simulink model "Auto_pilot"  (R2022a)
settings: Solver=VariableStepAuto  StartTime=0.0  StopTime=10  MaxStep=0.001  RelTol=1e-3
values from neighbouring files (symbols this model uses):
  a_phi1 = -1 * 0.5 * rho * Va^2 * S * b * C_pp * b / (2 * Va)    [Lateral_Autopilot.m]
  a_phi2 = 1 * 0.5 * rho * Va^2 * S * b * C_pa    [Lateral_Autopilot.m]
  k_d_phi = (2 * zeta_phi * w_n_phi - a_phi1) / a_phi2    [Lateral_Autopilot.m]
  k_i_phi = 1.5    [Lateral_Autopilot.m]
  k_p_phi = delta_a_max * sign(a_phi2) / e_max    [Lateral_Autopilot.m]
settings Model: Creator=ASUS  LastModifiedBy=Admin

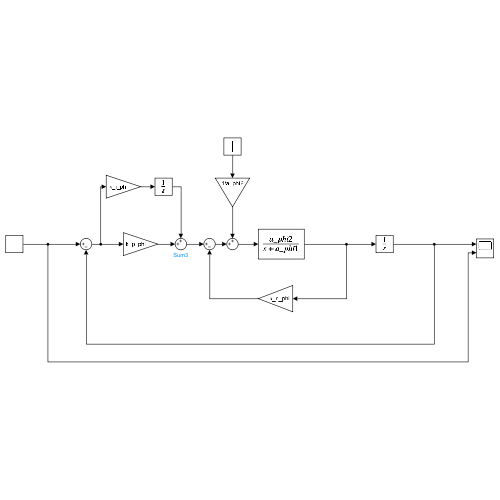
[thumbnail: Simulink's stored preview of the top-level diagram]
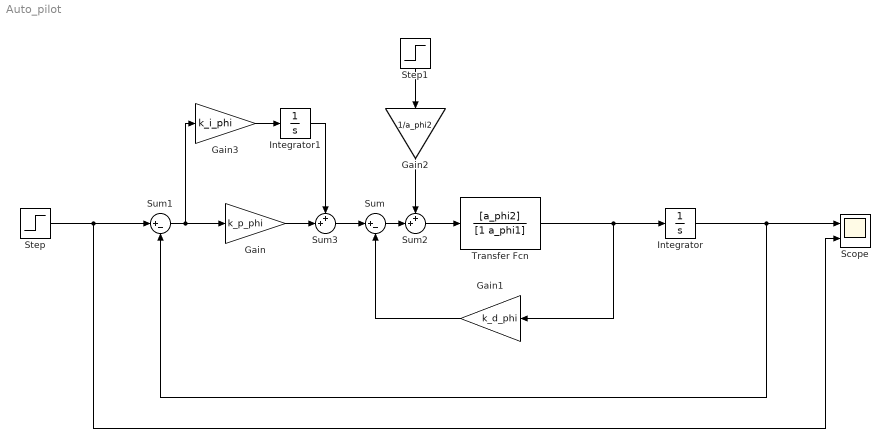
== system Auto_pilot ==
  Gain : Gain  Gain=k_p_phi
  Gain1 : Gain  Gain=k_d_phi
  Gain2 : Gain  Gain=1/a_phi2
  Gain3 : Gain  Gain=k_i_phi
  Integrator : Integrator
  Integrator1 : Integrator
  Scope : Scope  NumInputPorts=2
  Step : Step  SampleTime=0
  Step1 : Step  Time=0  After=0  SampleTime=0
  Sum : Sum  Inputs=|+-
  Sum1 : Sum  Inputs=|+-
  Sum2 : Sum  Inputs=++|
  Sum3 : Sum  Inputs=++|
  Transfer Fcn : TransferFcn  Numerator=[a_phi2]  Denominator=[1 a_phi1]
  wires:
  Integrator/1 -> Sum1/2, Scope/1
  Transfer Fcn/1 -> Gain1/1, Integrator/1
  Gain/1 -> Sum3/2
  Gain1/1 -> Sum/2
  Step/1 -> Scope/2, Sum1/1
  Sum1/1 -> Gain3/1, Gain/1
  Sum/1 -> Sum2/2
  Sum2/1 -> Transfer Fcn/1
  Gain2/1 -> Sum2/1
  Step1/1 -> Gain2/1
  Integrator1/1 -> Sum3/1
  Gain3/1 -> Integrator1/1
  Sum3/1 -> Sum/1
